simulink model "ex6"  (R2020a)
settings: Solver=VariableStepAuto  StartTime=0.0  StopTime=5  MaxStep=0.001  RelTol=1e-3
undefined symbols (not defined in the file): A, B, C, D, x0
settings Model: Creator=EREN  LastModifiedBy=EREN

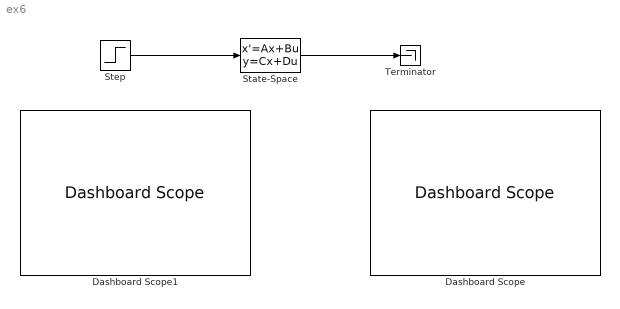
== system ex6 ==
  Dashboard Scope : DashboardScope
  Dashboard Scope1 : DashboardScope
  State-Space : StateSpace  A=A  B=B  C=C  D=D  InitialCondition=x0
  Step : Step  Time=0  Before=2  After=2  SampleTime=0
  Terminator : Terminator
  wires:
  Step/1 -> State-Space/1
  State-Space/1 -> Terminator/1
